simulink model "SB7_signal_done"  (R2024b)
settings: Solver=FixedStepDiscrete  StartTime=0.0  StopTime=10  FixedStep=0.05  RelTol=1e-3
settings Model: Creator=admin  LastModifiedBy=admin

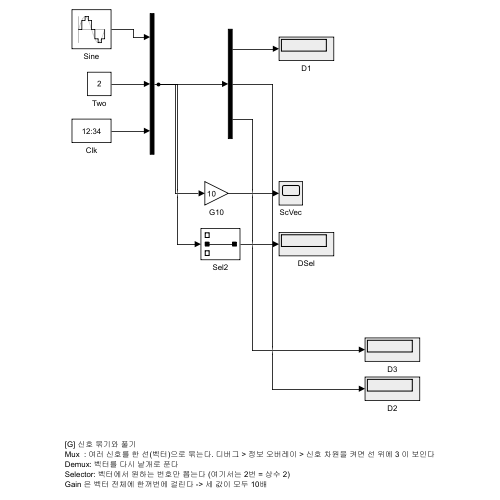
[thumbnail: Simulink's stored preview of the top-level diagram]
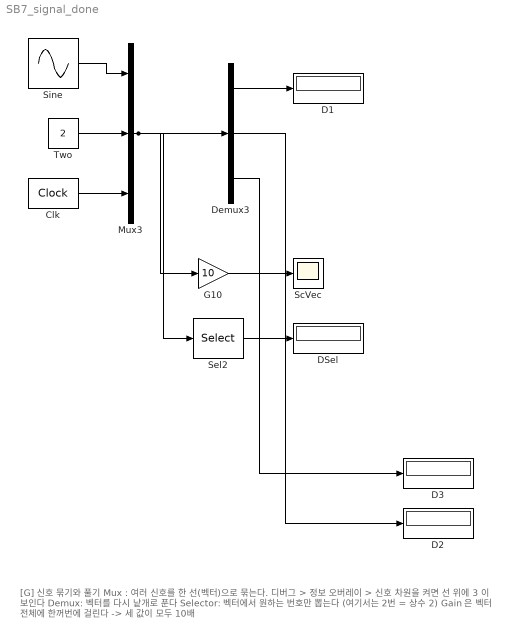
== system SB7_signal_done ==
  note: [G] 신호 묶기와 풀기
      | Mux  : 여러 신호를 한 선(벡터)으로 묶는다. 디버그 > 정보 오버레이 > 신호 차원을 켜면 선 위에 3 이 보인다
      | Demux: 벡터를 다시 낱개로 푼다
      | Selector: 벡터에서 원하는 번호만 뽑는다 (여기서는 2번 = 상수 2)
      | Gain 은 벡터 전체에 한꺼번에 걸린다 -> 세 값이 모두 10배
  Clk : DigitalClock  SampleTime=0.05
  D1 : Display
  D2 : Display
  D3 : Display
  DSel : Display
  Demux3 : Demux  Outputs=3
  G10 : Gain  Gain=10
  Mux3 : Mux  Inputs=3
  ScVec : Scope
  Sel2 : Selector  InputPortWidth=3  IndexOptions=Index vector (dialog)  Indices=2  OutputSizes=1
  Sine : Sin  SampleTime=0.05
  Two : Constant  Value=2
  wires:
  Demux3/1 -> D1/1
  Sine/1 -> Mux3/1
  Two/1 -> Mux3/2
  Mux3/1 -> Demux3/1, Sel2/1, G10/1
  Clk/1 -> Mux3/3
  G10/1 -> ScVec/1
  Sel2/1 -> DSel/1
  Demux3/3 -> D3/1
  Demux3/2 -> D2/1
